simulink model "simul6"  (R2014b)
settings: Solver=ode14x  StartTime=0.0  StopTime=100  FixedStep=dt  RelTol=1e-3
values from neighbouring files (symbols this model uses):
  ASg = 6    [LD6script.m]
  dt = 1e-3    (= 0.001)    [LD6script.m]
  dw_s = 2    [LD6script.m]
  n = 2    [LD6script.m]
libraries: dsparch4 x1, simulink x1
settings Model: Creator=Armands  LastModifiedBy=Armands

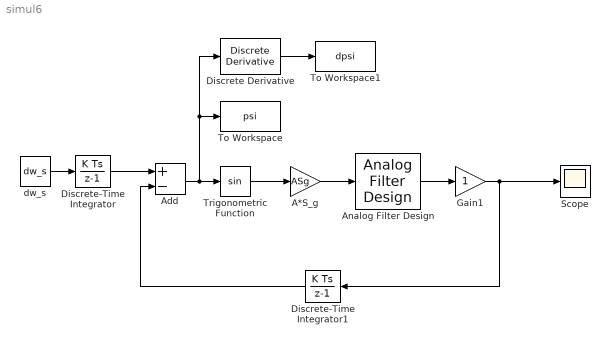
== system simul6 ==
  A*S_g : Gain  Gain=ASg  SampleTime=dt
  Add : Sum  Inputs=+-  SampleTime=dt
  Analog Filter Design : dsparch4/Analog Filter Design  method=Butterworth  filttype=Lowpass  N=n  Wlo=wn  Whi=80  Rp=2  Rs=40
  Discrete Derivative : simulink/Discrete/Discrete Derivative  gainval=1.0  ICPrevScaledInput=0.0  InputProcessing=Inherited  OutMin=[]  OutMax=[]  OutDataType=fixdt(1, 16)  OutScaling=2^-10  DoSatur=off
  Discrete-Time Integrator : DiscreteIntegrator  InitialConditionSetting=State (most efficient)  SampleTime=dt
  Discrete-Time Integrator1 : DiscreteIntegrator  InitialConditionSetting=State (most efficient)  SampleTime=dt
  Gain1 : Gain  SampleTime=dt
  Scope : Scope
      settings: YMin=-1  YMax=1.5  MaxDataPoints=10000
  To Workspace : ToWorkspace  VariableName=psi  SampleTime=-1
      settings: Save2DSignal=2-D array (concatenate along first dimension)
  To Workspace1 : ToWorkspace  VariableName=dpsi  SampleTime=-1
      settings: Save2DSignal=2-D array (concatenate along first dimension)
  Trigonometric Function : Trigonometry  OutputSignalType=real  SampleTime=dt
  dw_s : Constant  Value=dw_s  SampleTime=dt
  wires:
  Discrete-Time Integrator/1 -> Add/1
  Add/1 -> Discrete Derivative/1, To Workspace/1, Trigonometric Function/1
  Trigonometric Function/1 -> A*S_g/1
  A*S_g/1 -> Analog Filter Design/1
  Gain1/1 -> Scope/1, Discrete-Time Integrator1/1
  Discrete-Time Integrator1/1 -> Add/2
  dw_s/1 -> Discrete-Time Integrator/1
  Discrete Derivative/1 -> To Workspace1/1
  Analog Filter Design/1 -> Gain1/1
